simulink model "Ctrld_chopper"  (R2023b)
settings: Solver=ode45  StartTime=0.0  StopTime=0.3  MaxStep=1e-3  RelTol=1e-4
values from neighbouring files (symbols this model uses):
  E = 0    [TP_Hacheurs.m]
  L = 0.1    [TP_Hacheurs.m]
  R = 10    [TP_Hacheurs.m]
  T = 1/f    (= 0.002)    [TP_Hacheurs.m]
  U_Reference = -14    [TP_Hacheurs.m]
  Vdc = 50    [TP_Hacheurs.m]
libraries: spsCurrentMeasurementLib x3, spsMeanLib x2, spsDCVoltageSourceLib x2, simulink x1, spsDiodeLib x1, spsIGBTDiodeLib x1, spsSeriesRLCBranchLib x1, spsVoltageMeasurementLib x1, sps_lib x1
settings Model: Creator=Legrey  LastModifiedBy=Legrey

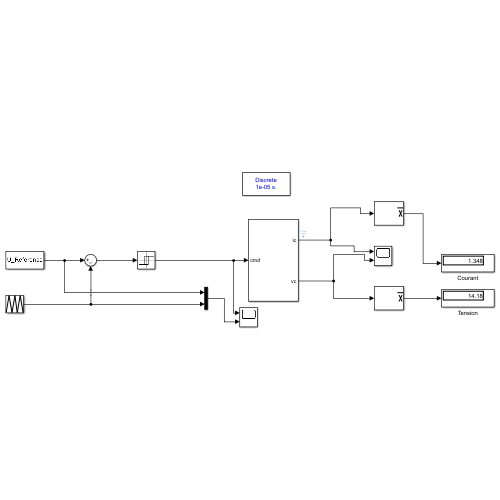
[thumbnail: Simulink's stored preview of the top-level diagram]
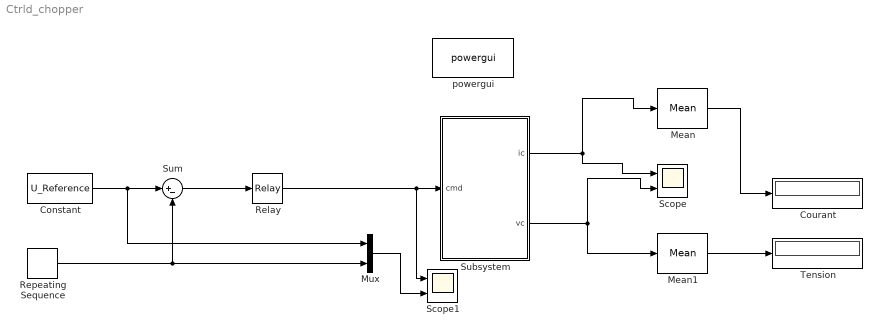
== system Ctrld_chopper ==
  Constant : Constant  Value=U_Reference
  Courant : Display
  Mean : spsMeanLib/Mean  Freq=f  Vinit=0  Ts=0
  Mean1 : spsMeanLib/Mean  Freq=f  Vinit=0  Ts=0
  Mux : Mux  Inputs=2
  Relay : Relay  OnSwitchValue=0  OffSwitchValue=0
  Repeating Sequence : simulink/Sources/Repeating Sequence  rep_seq_t=[0 1/2 1]*T  rep_seq_y=[0 Vdc 0]
  Scope : Scope  NumInputPorts=2
  Scope1 : Scope  NumInputPorts=2
  Subsystem : Subsystem
  Sum : Sum  Inputs=|+-
  Tension : Display
  powergui : sps_lib/powergui  Priority=1  SimulationMode=Discrete  SampleTime=1e-005  frequency=60  Iterations=50  frequencyindice=0  Pbase=100e6  ErrMax=1e-4  UnitsV=kV  UnitsW=MW  buscounter=0  FunctionMessages=off  echomessages=off  EnableUseOfTLC=off  CurrentSourceSwitches=off  DisableSnubberDevices=off  DisableRonSwitches=off  DisableVfSwitches=off  DisplayEquations=off  AutomaticDiscreteSolvers=off  SolverType=Tustin/Backward Euler (TBE)  Interpol=off  ExternalGateDelay=off  methode=off  Ts=100  x0status=blocks  SPID=on  SwTol=0  HookPort=off  NonlinearTolerance=1e-4  nMaxIteration=100  ContinueOnMaxIteration=off  RestoreLinks=warning  ResistiveCurrentMeasurement=off  Frange=[0:2:500]  Ylog=off  Xlog=on  ShowGrid=off  save=off  variable=ZData  structure=0  ZoomFFT=off  StartTime=0.0  cycles=1  DisplayStyle=1  fundamental=60  FreqAxis=off  MaxFrequency=1000  frequencyindicesteady=1  RmsSteady=1  display=off
  wires:
  Subsystem/1(ic) -> Mean/1, Scope/1
  Subsystem/2(vc) -> Scope/2, Mean1/1
  Mean1/1 -> Tension/1
  Mean/1 -> Courant/1
  Repeating Sequence/1 -> Sum/2, Mux/2
  Mux/1 -> Scope1/2
  Sum/1 -> Relay/1
  Relay/1 -> Subsystem/1(cmd), Scope1/1
  Constant/1 -> Mux/1, Sum/1

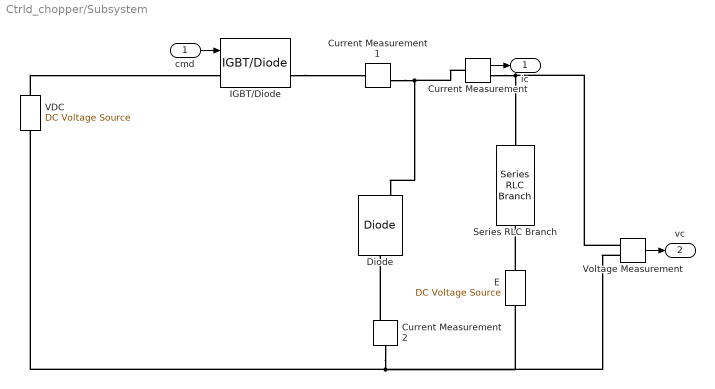
== system Ctrld_chopper/Subsystem ==
  cmd : Inport
  Current Measurement : spsCurrentMeasurementLib/Current Measurement  PhasorSimulation=off  OutputType=Complex  PSBequivalent=0
  Current Measurement1 : spsCurrentMeasurementLib/Current Measurement  PhasorSimulation=off  OutputType=Complex  PSBequivalent=0
  Current Measurement2 : spsCurrentMeasurementLib/Current Measurement  PhasorSimulation=off  OutputType=Complex  PSBequivalent=0
  Diode : spsDiodeLib/Diode  Ron=0.001  Lon=0  Vf=0.8  IC=0  UseSnubber=0  Rs=500  Cs=250e-9  Measurements=on
  E : spsDCVoltageSourceLib/DC Voltage Source  Amplitude=E  Measurements=None
  IGBT/Diode : spsIGBTDiodeLib/IGBT//Diode  Ron=1e-3  Rs=1e5  Cs=inf  Measurements=on
  Series RLC Branch : spsSeriesRLCBranchLib/Series RLC Branch  LConnTagsString=__new0  RConnTagsString=__new0  BranchType=RL  Resistance=R  Inductance=L  SetiL0=off  InitialCurrent=0  Capacitance=0  Setx0=off  InitialVoltage=0  Measurements=None
  VDC : spsDCVoltageSourceLib/DC Voltage Source  Amplitude=Vdc  Measurements=None
  Voltage Measurement : spsVoltageMeasurementLib/Voltage Measurement  PhasorSimulation=off  OutputType=Complex  PSBequivalent=0
  ic : Outport
  vc : Outport  Port=2
  wires:
  cmd/1 -> IGBT/Diode/1
  Voltage Measurement/1 -> vc/1
  Current Measurement/1 -> ic/1
  connections:
  Current Measurement1/RConn1 -- Diode/RConn1 -- Current Measurement/LConn1
  Current Measurement/RConn1 -- Series RLC Branch/LConn1 -- Voltage Measurement/LConn1
  Current Measurement2/LConn1 -- Voltage Measurement/LConn2 -- E/LConn1 -- VDC/LConn1
  E/RConn1 -- Series RLC Branch/RConn1
  VDC/RConn1 -- IGBT/Diode/LConn1
  IGBT/Diode/RConn1 -- Current Measurement1/LConn1
  Current Measurement2/RConn1 -- Diode/LConn1
